simulink model "exp1"  (R2013a)
settings: Solver=ode45  StartTime=0.0  StopTime=5  RelTol=1e-3
undefined symbols (not defined in the file): National_Instruments, PCI, pin
libraries: simulink x5, rtwinlib x4
settings Model: Creator=abc  LastModifiedBy=CC LAB

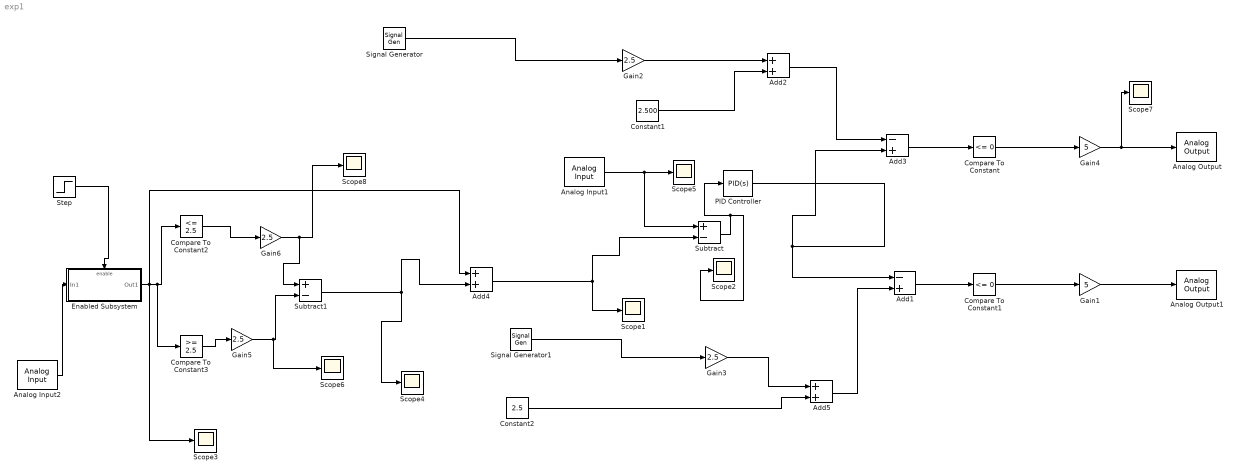
== system exp1 ==
  Add1 : Sum  Inputs=-+
  Add2 : Sum
  Add3 : Sum  Inputs=-+
  Add4 : Sum
  Add5 : Sum
  Analog Input1 : rtwinlib/Analog Input  SampleTime=0.001  MaxMissedTicks=10000  ShowMissedTicks=off  YieldWhenWaiting=off  DrvName=National_Instruments/PCI-6221_37-pin  DrvAddress=0  DrvOptions=[0 3 0 0 0]  Channels=1  RangeMode=1  VoltRange=1  DataType=1
      settings: AttributesFormatString=National Instruments\nPCI-6221 37-pin [0h]
  Analog Input2 : rtwinlib/Analog Input  SampleTime=0.001  MaxMissedTicks=10000  ShowMissedTicks=off  YieldWhenWaiting=off  DrvName=National_Instruments/PCI-6221_37-pin  DrvAddress=0  DrvOptions=[0 3 0 0 0]  Channels=1  RangeMode=1  VoltRange=1  DataType=1
      settings: AttributesFormatString=National Instruments\nPCI-6221 37-pin [0h]
  Analog Output : rtwinlib/Analog Output  SampleTime=0.001  MaxMissedTicks=10000  ShowMissedTicks=off  YieldWhenWaiting=off  DrvName=National_Instruments/PCI-6221_37-pin  DrvAddress=0  DrvOptions=[0 3 0 0 0]  Channels=1  RangeMode=1  VoltRange=1  InitialValue=0  FinalValue=0
      settings: AttributesFormatString=National Instruments\nPCI-6221 37-pin [0h]
  Analog Output1 : rtwinlib/Analog Output  SampleTime=0.001  MaxMissedTicks=10000  ShowMissedTicks=off  YieldWhenWaiting=off  DrvName=National_Instruments/PCI-6221_37-pin  DrvAddress=0  DrvOptions=[0 3 0 0 0]  Channels=2  RangeMode=1  VoltRange=1  InitialValue=0  FinalValue=0
      settings: AttributesFormatString=National Instruments\nPCI-6221 37-pin [0h]
  Compare To Constant : simulink/Logic and Bit Operations/Compare To Constant  relop=<=  const=0  OutDataTypeStr=uint8
  Compare To Constant1 : simulink/Logic and Bit Operations/Compare To Constant  relop=<=  const=0  OutDataTypeStr=uint8
  Compare To Constant2 : simulink/Logic and Bit Operations/Compare To Constant  relop=<=  const=2.5  OutDataTypeStr=boolean
  Compare To Constant3 : simulink/Logic and Bit Operations/Compare To Constant  relop=>=  const=2.5  OutDataTypeStr=boolean
  Constant1 : Constant  Value=2.500
  Constant2 : Constant  Value=2.5
  Enabled Subsystem : Subsystem  TreatAsAtomicUnit=on
  Gain1 : Gain  Gain=5  ParamMin=0  OutMin=0  RndMeth=Ceiling  OutDataTypeStr=Inherit: Same as input
  Gain2 : Gain  Gain=2.5  ParamMin=0  OutMin=0  RndMeth=Ceiling  OutDataTypeStr=Inherit: Same as input
  Gain3 : Gain  Gain=2.5  ParamMin=0  OutMin=0  RndMeth=Ceiling  OutDataTypeStr=Inherit: Same as input
  Gain4 : Gain  Gain=5  ParamMin=0  OutMin=0  RndMeth=Ceiling  OutDataTypeStr=Inherit: Same as input
  Gain5 : Gain  Gain=2.5  ParamMin=0  OutMin=0  OutDataTypeStr=double  RndMeth=Ceiling
  Gain6 : Gain  Gain=2.5  ParamMin=0  OutMin=0  OutDataTypeStr=double  RndMeth=Ceiling
  PID Controller : simulink/Continuous/PID Controller  Controller=PID  TimeDomain=Continuous-time  SampleTime=1  IntegratorMethod=Forward Euler  FilterMethod=Forward Euler  Form=Parallel  P=60  I=1  D=1  N=100  InitialConditionSource=internal  InitialConditionForIntegrator=0  InitialConditionForFilter=0  ExternalReset=none  LimitOutput=off  UpperSaturationLimit=inf  LowerSaturationLimit=-inf  LinearizeAsGain=on  AntiWindupMode=none  Kb=1  TrackingMode=off  Kt=1  PParamMin=[]  PParamMax=[]  IParamMin=[]  IParamMax=[]  DParamMin=[]  DParamMax=[]  NParamMin=[]  NParamMax=[]  KbParamMin=[]  KbParamMax=[]  KtParamMin=[]  KtParamMax=[]  POutMin=[]  POutMax=[]  IOutMin=[]  IOutMax=[]  DOutMin=[]  DOutMax=[]  NOutMin=[]  NOutMax=[]  KbOutMin=[]  KbOutMax=[]  KtOutMin=[]  KtOutMax=[]  IntegratorOutMin=[]  IntegratorOutMax=[]  FilterOutMin=[]  FilterOutMax=[]  SumOutMin=[]  SumOutMax=[]  SumI1OutMin=[]  SumI1OutMax=[]  SumI2OutMin=[]  SumI2OutMax=[]  SumI3OutMin=[]  SumI3OutMax=[]  SumDOutMin=[]  SumDOutMax=[]  SaturationOutMin=[]  SaturationOutMax=[]  IntegratorContinuousStateAttributes=''  IntegratorStateMustResolveToSignalObject=off  IntegratorRTWStateStorageClass=Auto  FilterContinuousStateAttributes=''  FilterStateMustResolveToSignalObject=off  FilterRTWStateStorageClass=Auto
  Scope{1..8} (8 alike) : Scope
      Scope1 settings: TimeRange=10  YMin=-3  YMax=3.5  MaxDataPoints=1000000
      Scope2 settings: TimeRange=10  YMin=-3  YMax=3.5  MaxDataPoints=1000000
      Scope3 settings: TimeRange=10  YMin=-3  YMax=3.5  SaveName=ScopeData2  MaxDataPoints=1000000
      Scope4 settings: TimeRange=10  YMin=-3  YMax=3.5  SaveName=ScopeData3  MaxDataPoints=1000000
      Scope5 settings: TimeRange=10  YMin=-3  YMax=3.5  SaveName=ScopeData4  MaxDataPoints=1000000
      Scope6 settings: TimeRange=10  YMin=-3  YMax=3.5  SaveName=ScopeData5  MaxDataPoints=1000000
      Scope7 settings: TimeRange=10  YMin=-3  YMax=3.5  SaveName=ScopeData6  MaxDataPoints=1000000
      Scope8 settings: TimeRange=10  YMin=-3  YMax=3.5  SaveName=ScopeData7  MaxDataPoints=1000000
  Signal Generator : SignalGenerator  WaveForm=sawtooth  Frequency=200
  Signal Generator1 : SignalGenerator  WaveForm=sawtooth  Frequency=1000
  Step : Step  Time=0.01  Before=1  After=0  SampleTime=0
  Subtract : Sum  Inputs=+-
  Subtract1 : Sum  Inputs=+-
  wires:
  Add3/1 -> Compare To Constant/1
  Compare To Constant/1 -> Gain4/1
  Gain4/1 -> Scope7/1, Analog Output/1
  Add1/1 -> Compare To Constant1/1
  Compare To Constant1/1 -> Gain1/1
  Gain1/1 -> Analog Output1/1
  Add2/1 -> Add3/1
  Gain3/1 -> Add5/1
  Constant2/1 -> Add5/2
  Add5/1 -> Add1/2
  PID Controller/1 -> Add3/2, Add1/1
  Analog Input1/1 -> Scope5/1, Subtract/1
  Constant1/1 -> Add2/2
  Gain2/1 -> Add2/1
  Signal Generator/1 -> Gain2/1
  Signal Generator1/1 -> Gain3/1
  Step/1 -> Enabled Subsystem/Enable
  Analog Input2/1 -> Enabled Subsystem/1(In1)
  Add4/1 -> Scope1/1, Subtract/2
  Subtract/1 -> PID Controller/1, Scope2/1
  Enabled Subsystem/1(Out1) -> Scope3/1, Add4/1, Compare To Constant2/1, Compare To Constant3/1
  Subtract1/1 -> Add4/2, Scope4/1
  Compare To Constant3/1 -> Gain5/1
  Gain5/1 -> Scope6/1, Subtract1/2
  Compare To Constant2/1 -> Gain6/1
  Gain6/1 -> Subtract1/1, Scope8/1

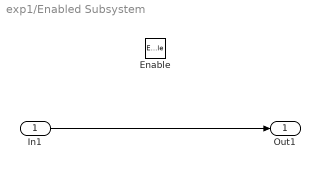
== system exp1/Enabled Subsystem ==
  In1 : Inport
  Enable : EnablePort
  Out1 : Outport
  wires:
  In1/1 -> Out1/1
